simulink model "Super1NoActions"  (Simulink 9.0)
settings: Solver=ode45  StartTime=0.0  StopTime=10.0  RelTol=1e-3  EnableMultiTasking=on
settings Model: SuppressorTable=22 serialization::archive 11 0 6 0 0 0 0 0  Creator=scaife  LastModifiedBy=ktrinh  ExtModeAutoUpdateStatusClock=off
settings DataIOCC: LimitDataPoints=on  SignalLoggingSaveFormat=ModelDataLogs  SignalLoggingName=sigsOut
settings DebuggingCC: SaveWithParameterizedLinksMsg=none  SignalResolutionControl=TryResolveAllWithWarning  MultiTaskDSMMsg=warning  MultiTaskCondExecSysMsg=none
settings HardwareCC: TargetUnknown=on
settings SFSimCC: SimParseCustomCode=off
settings GRTTargetCC: CombineOutputUpdateFcns=off  GRTInterface=on

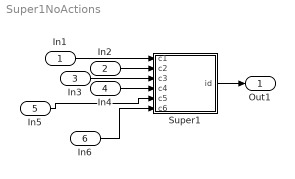
== system Super1NoActions ==
  In1 : Inport  OutDataTypeStr=boolean
  In2 : Inport  Port=2  OutDataTypeStr=boolean
  In3 : Inport  Port=3  OutDataTypeStr=boolean
  In4 : Inport  Port=4  OutDataTypeStr=boolean
  In5 : Inport  Port=5  OutDataTypeStr=boolean
  In6 : Inport  Port=6  OutDataTypeStr=boolean
  Super1 : Stateflow chart  TreatAsAtomicUnit=on
  Out1 : Outport
  wires:
  Super1/1(id) -> Out1/1
  In1/1 -> Super1/1(c1)
  In2/1 -> Super1/2(c2)
  In3/1 -> Super1/3(c3)
  In4/1 -> Super1/4(c4)
  In5/1 -> Super1/5(c5)
  In6/1 -> Super1/6(c6)

== stateflow chart Super1 ==
  state A
    en : id = 1;
  state B
    en : id = 5;
  state C
    state C1
      en : id = 3;
    state C2
      en : id = 4;
    (default) -> C1
    C2 -> C1 [order 2] : [c5]
    C1 -> C2 [order 2] : [c5]
  state D
    en : id = 2;
  (default) -> A
  C1 -> B [order 1] : [c2]
  (junction 19) -> C1 [order 1] : [c1]
  A -> (junction 19) : [c3]
  (junction 19) -> D [order 2] : [c5]
  B -> C2 : [c3]
  D -> A : [c6]
  (junction 20) -> A [order 2] : [c2]
  C2 -> (junction 20) [order 1] : [c4]
  (junction 20) -> D [order 1] : [c4]
  data: c1 input boolean; c2 input boolean; c3 input boolean; c4 input boolean; c5 input boolean; c6 input boolean; id output double
